simulink model "firmwareTestValues"  (R2024a)
settings: Solver=VariableStepAuto  StartTime=0.0  StopTime=10  RelTol=1e-3
undefined symbols (not defined in the file or in its folder): mes_mag, mes_ss, omega, ref_mag, ref_ss, use_sun_sensor
settings Model: Creator=joshu  LastModifiedBy=joshu
settings OptimizationCC: DefaultParameterBehavior=Inlined  UseDivisionForNetSlopeComputation=on  GainParamInheritBuiltInType=on  UseFloatMulNetSlope=on  InlineInvariantSignals=on  PassReuseOutputArgsAs=Individual arguments  ZeroExternalMemoryAtStartup=off  ZeroInternalMemoryAtStartup=off  NoFixptDivByZeroProtection=on  EfficientFloat2IntCast=on  LifeSpan=1  OptimizeBlockOrder=speed  DifferentSizesBufferReuse=on  EfficientTunableParamExpr=on
settings DebuggingCC: ParameterTunabilityLossMsg=error
settings HardwareCC: ProdBitPerPointer=32  ProdBitPerSizeT=32  ProdBitPerPtrDiffT=32  ProdLargestAtomicInteger=Long  ProdLargestAtomicFloat=Double  ProdWordSize=32  ProdLongLongMode=on  ProdHWDeviceType=ARM Compatible->ARM Cortex-R
settings SFSimCC: MATLABDynamicMemAlloc=off
settings RTWCC: Description=Embedded Coder  SystemTargetFile=ert.tlc  GenCodeOnly=on  TemplateMakefile=ert_default_tmf
settings CodeAppCC: ForceParamTrailComments=on  IgnoreCustomStorageClasses=off  OperatorAnnotations=on  SimulinkDataObjDesc=on  SFDataObjDesc=on  CustomSymbolStrGlobalVar=rt$N$M  CustomSymbolStrType=$N$M  CustomSymbolStrFcn=$N$M$F  CustomSymbolStrMacro=$N$M  InsertBlockDesc=on
settings ERTTargetCC: TargetLangStandard=C99 (ISO)  GenerateSampleERTMain=on  IncludeMdlTerminateFcn=off  CombineSignalStateStructs=on  SupportAbsoluteTime=off  SupportComplex=off  SupportContinuousTime=on  InlinedParameterPlacement=NonHierarchical  ERTCustomFileTemplate=example_file_process.tlc  ERTFilePackagingFormat=CompactWithDataFile

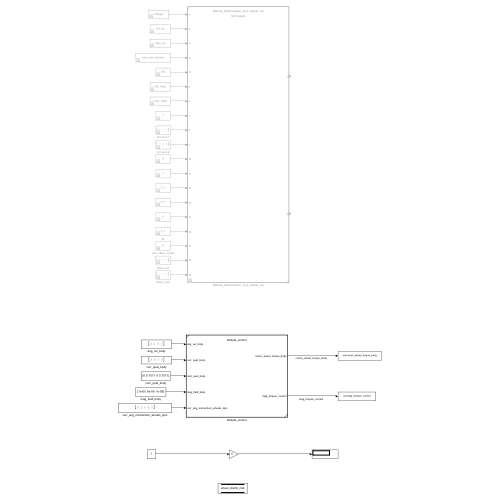
[thumbnail: Simulink's stored preview of the top-level diagram]
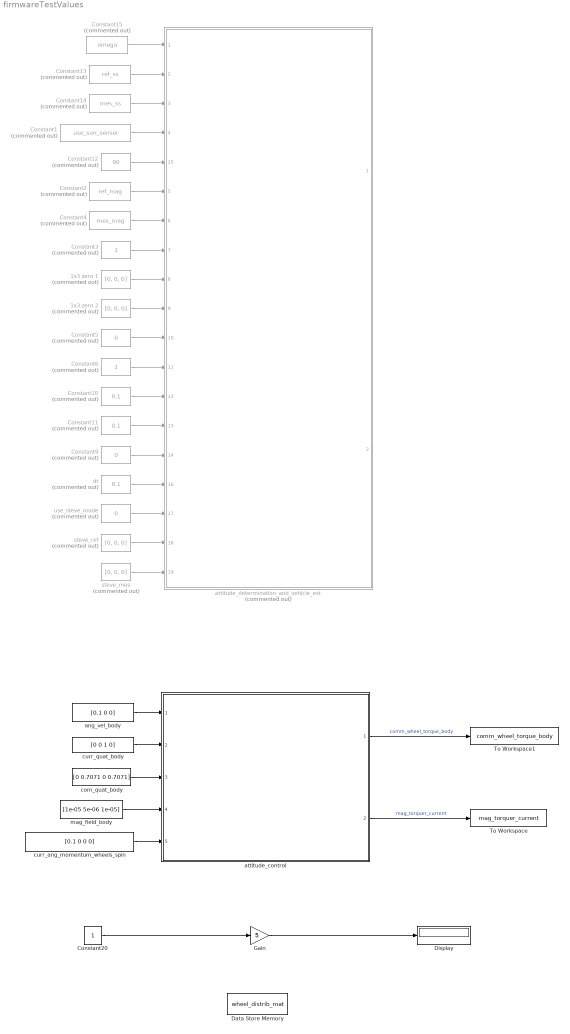
== system firmwareTestValues ==
  1x3 zero 1 : Constant  Commented=on  Value=[0, 0, 0]
  1x3 zero 2 : Constant  Commented=on  Value=[0, 0, 0]
  Constant1 : Constant  Commented=on  Value=use_sun_sensor
  Constant10 : Constant  Commented=on  Value=0.1
  Constant11 : Constant  Commented=on  Value=0.1
  Constant12 : Constant  Commented=on  Value=90
  Constant13 : Constant  Commented=on  Value=ref_ss
  Constant14 : Constant  Commented=on  Value=mes_ss
  Constant15 : Constant  Commented=on  Value=omega
  Constant2 : Constant  Commented=on  Value=ref_mag
  Constant20 : Constant
  Constant3 : Constant  Commented=on  OutDataTypeStr=boolean
  Constant4 : Constant  Commented=on  Value=mes_mag
  Constant5 : Constant  Commented=on  Value=0  OutDataTypeStr=boolean
  Constant6 : Constant  Commented=on  OutDataTypeStr=boolean
  Constant9 : Constant  Commented=on  Value=0
  Data Store Memory : DataStoreMemory  DataStoreName=wheel_distrib_mat  WriteAfterWriteMsg=warning  InitialValue=[0.5736 0.5736 0.5736 0.5736 ; 0.8192 -0.8192 0 0 ; 0 0 0.8192 -0.8192]  ShowAdditionalParam=off
  Display : Display
  Gain : Gain  Gain=5
  To Workspace : ToWorkspace  VariableName=mag_torquer_current  SaveFormat=Timeseries  SampleTime=-1
  To Workspace1 : ToWorkspace  VariableName=comm_wheel_torque_body  SaveFormat=Timeseries  SampleTime=-1
  ang_vel_body : Constant  Value=[0.1 0 0]
  attitude_control : Subsystem  TreatAsAtomicUnit=on  ReferencedSubsystem=attitude_control
  attitude_determination_and_vehicle_est : Subsystem  Commented=on  TreatAsAtomicUnit=on  SystemSampleTime=0.1  ReferencedSubsystem=attitude_determination_and_vehicle_est
      settings: PortSchema="{\"entries\":[{\"content\":{\"sides\":[{\"content\":{\"connectorIds\":[\"In1\",\"In2\",\"In3\",\"In4\",\"In15\",\"In5\",\"In6\",\"In7\",\"In8\",\"In9\",\"In10\",\"In11\",\"In12\",\"In13\",\"In14\",\"In16\",\"In17\",\"In18\",\"In19\"]},\"type\":\"ConnectorPlacement.EquallySpacedRectSide\",\"uuid\":\"3b22937b-158d-42bc-8266-221df4d5bb4f\"},{\"content\":{\"connectorIds\":[\"Out1\",\"Out2\"],\"side\":\"RIGHT\"},\"type\":\"ConnectorPlacement.EquallySpacedRectSide\",\"uuid\":\"2d7976b0-5d09-4ece-a5b5-6f5d6f0d46dd\"},{\"content\":{\"side\":\"TOP\"},\"type\":\"ConnectorPlacement.EquallySpacedRectSide\",\"uuid\":\"411abe81-91ab-4e83-a0ca-8600290f09f5\"}]},\"type\":\"ConnectorPlacement.EquallySpacedConnector\",\"uuid\":\"dff24d4c-a30b-41c1-92cc-a12930c50369\"}],\"packageUris\":[\"http://schema.mathworks.com/mf0/Connector/R2020b\"],\"version\":\"1.0\"}"
  com_quat_body : Constant  Value=[0 0.7071 0 0.7071]
  curr_ang_momentum_wheels_spin : Constant  Value=[0.1 0 0 0]
  curr_quat_body : Constant  Value=[0 0 1 0]
  dt : Constant  Commented=on  Value=0.1
  mag_field_body : Constant  Value=[1e-05 5e-06 1e-05]
  steve_mes : Constant  Commented=on  Value=[0, 0, 0]
  steve_ref : Constant  Commented=on  Value=[0, 0, 0]
  use_steve_mode : Constant  Commented=on  Value=0  OutDataTypeStr=boolean
  wires:
  Constant12/1 -> attitude_determination_and_vehicle_est/15
  Constant11/1 -> attitude_determination_and_vehicle_est/13
  Constant13/1 -> attitude_determination_and_vehicle_est/2
  Constant2/1 -> attitude_determination_and_vehicle_est/5
  Constant14/1 -> attitude_determination_and_vehicle_est/3
  Constant4/1 -> attitude_determination_and_vehicle_est/6
  Constant15/1 -> attitude_determination_and_vehicle_est/1
  dt/1 -> attitude_determination_and_vehicle_est/16
  Constant6/1 -> attitude_determination_and_vehicle_est/11
  1x3 zero 2/1 -> attitude_determination_and_vehicle_est/9
  steve_ref/1 -> attitude_determination_and_vehicle_est/18
  steve_mes/1 -> attitude_determination_and_vehicle_est/19
  Constant3/1 -> attitude_determination_and_vehicle_est/7
  Constant9/1 -> attitude_determination_and_vehicle_est/14
  use_steve_mode/1 -> attitude_determination_and_vehicle_est/17
  1x3 zero 1/1 -> attitude_determination_and_vehicle_est/8
  Constant10/1 -> attitude_determination_and_vehicle_est/12
  Constant5/1 -> attitude_determination_and_vehicle_est/10
  Constant1/1 -> attitude_determination_and_vehicle_est/4
  curr_ang_momentum_wheels_spin/1 -> attitude_control/5
  mag_field_body/1 -> attitude_control/4
  com_quat_body/1 -> attitude_control/3
  curr_quat_body/1 -> attitude_control/2
  ang_vel_body/1 -> attitude_control/1
  Constant20/1 -> Gain/1
  Gain/1 -> Display/1
  attitude_control/1 -> To Workspace1/1  "comm_wheel_torque_body"
  attitude_control/2 -> To Workspace/1  "mag_torquer_current"
